simulink subsystem "TrqDemController"  (R2020b)
settings: Solver=VariableStepAuto  StartTime=0.0  StopTime=10.0  RelTol=1e-3
undefined symbols (not defined in the file): brkTrqMax, brkTrqMGU, TrqICMax, TrqMax, TrqMGUMax
libraries: eeGeneralControl x2
settings Model: Creator=francescoprignoli  LastModifiedBy=francescoprignoli

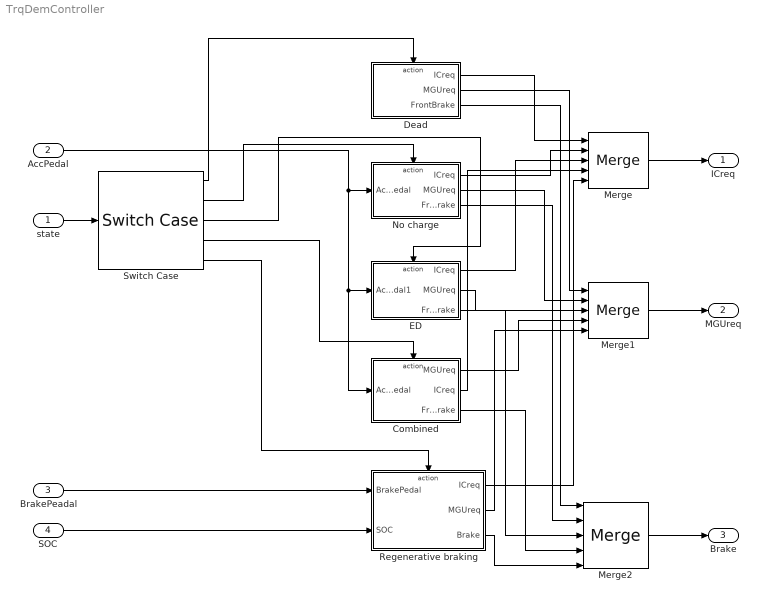
== system TrqDemController ==
  state : Inport
  AccPedal : Inport  Port=2
  BrakePeadal : Inport  Port=3
  SOC : Inport  Port=4
  Combined : Subsystem  TreatAsAtomicUnit=on
  Dead : Subsystem  TreatAsAtomicUnit=on
  ED : Subsystem  TreatAsAtomicUnit=on
  Merge : Merge  Inputs=5
  Merge1 : Merge  Inputs=5
  Merge2 : Merge  Inputs=5
  No charge : Subsystem  TreatAsAtomicUnit=on
  Regenerative braking : Subsystem  TreatAsAtomicUnit=on
  Switch Case : SwitchCase  CaseConditions={0,1,2,3,4}  ShowDefaultCase=off
  ICreq : Outport
  MGUreq : Outport  Port=2
  Brake : Outport  Port=3
  wires:
  Switch Case/1 -> Dead/Action
  ED/1(ICreq) -> Merge/3
  Merge1/1 -> MGUreq/1
  Regenerative braking/2(MGUreq) -> Merge1/5
  Dead/1(ICreq) -> Merge/1
  Regenerative braking/1(ICreq) -> Merge/5
  state/1 -> Switch Case/1
  Switch Case/5 -> Regenerative braking/Action
  AccPedal/1 -> ED/1(AccPedal1), Combined/1(AccPedal), No charge/1(AccPedal)
  Switch Case/4 -> Combined/Action
  Switch Case/3 -> ED/Action
  ED/2(MGUreq) -> Merge1/3
  SOC/1 -> Regenerative braking/2(SOC)
  Combined/1(MGUreq) -> Merge1/4
  No charge/2(MGUreq) -> Merge1/2
  Dead/2(MGUreq) -> Merge1/1
  Combined/2(ICreq) -> Merge/4
  Merge/1 -> ICreq/1
  Switch Case/2 -> No charge/Action
  No charge/1(ICreq) -> Merge/2
  BrakePeadal/1 -> Regenerative braking/1(BrakePedal)
  Dead/3(FrontBrake) -> Merge2/1
  No charge/3(FrontBrake) -> Merge2/2
  ED/3(FrontBrake) -> Merge2/3
  Combined/3(FrontBrake) -> Merge2/4
  Regenerative braking/3(Brake) -> Merge2/5
  Merge2/1 -> Brake/1

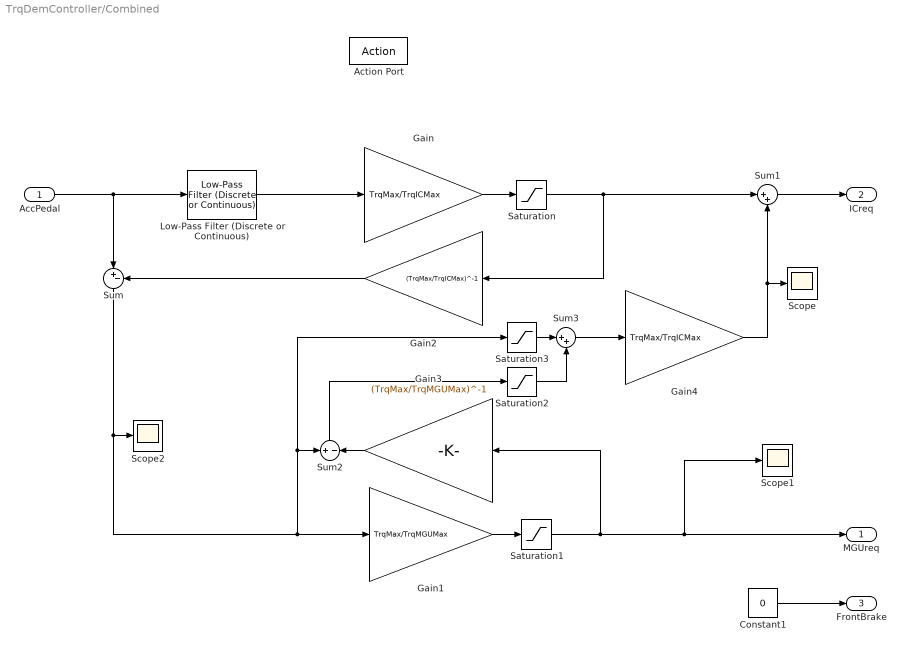
== system TrqDemController/Combined ==
  AccPedal : Inport
  Action Port : ActionPort
  Constant1 : Constant  Value=0
  Gain : Gain  Gain=TrqMax/TrqICMax
  Gain1 : Gain  Gain=TrqMax/TrqMGUMax
  Gain2 : Gain  Gain=(TrqMax/TrqICMax)^-1
  Gain3 : Gain  Gain=(TrqMax/TrqMGUMax)^-1
  Gain4 : Gain  Gain=TrqMax/TrqICMax
  Low-Pass Filter (Discrete or Continuous) : eeGeneralControl/Low-Pass Filter (Discrete or Continuous)  K=1  T=2  B=inf  A=-inf  init_option=Inherited from block input  x0=0  Ts=-1
  Saturation : Saturate  UpperLimit=1  LowerLimit=0
  Saturation1 : Saturate  UpperLimit=1  LowerLimit=0
  Saturation2 : Saturate  UpperLimit=1  LowerLimit=0
  Saturation3 : Saturate  UpperLimit=0  LowerLimit=-1
  Scope : Scope
  Scope1 : Scope
  Scope2 : Scope
  Sum : Sum  Inputs=|+-
  Sum1 : Sum  Inputs=|++
  Sum2 : Sum  Inputs=+|-
  Sum3 : Sum  Inputs=|++
  MGUreq : Outport
  ICreq : Outport  Port=2
  FrontBrake : Outport  Port=3
  wires:
  Gain4/1 -> Sum1/2, Scope/1
  Constant1/1 -> FrontBrake/1
  Saturation2/1 -> Sum3/2
  Sum3/1 -> Gain4/1
  Saturation3/1 -> Sum3/1
  Sum2/1 -> Saturation2/1
  Sum1/1 -> ICreq/1
  AccPedal/1 -> Sum/1, Low-Pass Filter (Discrete or Continuous)/1
  Sum/1 -> Sum2/1, Saturation3/1, Gain1/1, Scope2/1
  Gain/1 -> Saturation/1
  Gain1/1 -> Saturation1/1
  Saturation/1 -> Gain2/1, Sum1/1
  Saturation1/1 -> Gain3/1, MGUreq/1, Scope1/1
  Low-Pass Filter (Discrete or Continuous)/1 -> Gain/1
  Gain3/1 -> Sum2/2
  Gain2/1 -> Sum/2

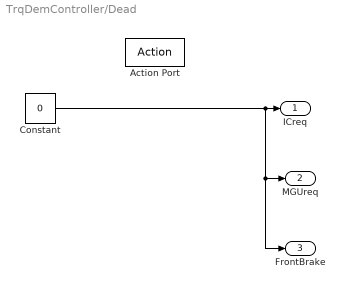
== system TrqDemController/Dead ==
  Action Port : ActionPort
  Constant : Constant  Value=0
  ICreq : Outport
  MGUreq : Outport  Port=2
  FrontBrake : Outport  Port=3
  wires:
  Constant/1 -> MGUreq/1, FrontBrake/1, ICreq/1

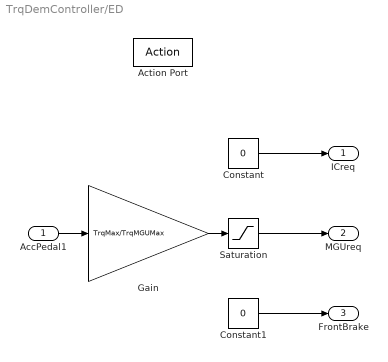
== system TrqDemController/ED ==
  AccPedal1 : Inport
  Action Port : ActionPort
  Constant : Constant  Value=0
  Constant1 : Constant  Value=0
  Gain : Gain  Gain=TrqMax/TrqMGUMax
  Saturation : Saturate  UpperLimit=1  LowerLimit=0
  ICreq : Outport
  MGUreq : Outport  Port=2
  FrontBrake : Outport  Port=3
  wires:
  Constant1/1 -> FrontBrake/1
  Constant/1 -> ICreq/1
  AccPedal1/1 -> Gain/1
  Gain/1 -> Saturation/1
  Saturation/1 -> MGUreq/1

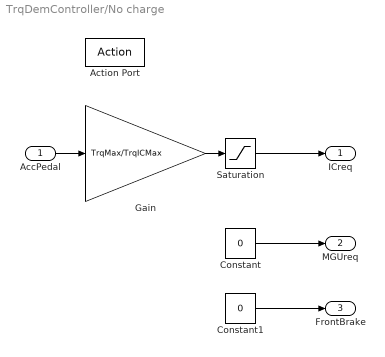
== system TrqDemController/No charge ==
  AccPedal : Inport
  Action Port : ActionPort
  Constant : Constant  Value=0
  Constant1 : Constant  Value=0
  Gain : Gain  Gain=TrqMax/TrqICMax
  Saturation : Saturate  UpperLimit=1  LowerLimit=0
  ICreq : Outport
  MGUreq : Outport  Port=2
  FrontBrake : Outport  Port=3
  wires:
  Constant1/1 -> FrontBrake/1
  Gain/1 -> Saturation/1
  AccPedal/1 -> Gain/1
  Saturation/1 -> ICreq/1
  Constant/1 -> MGUreq/1

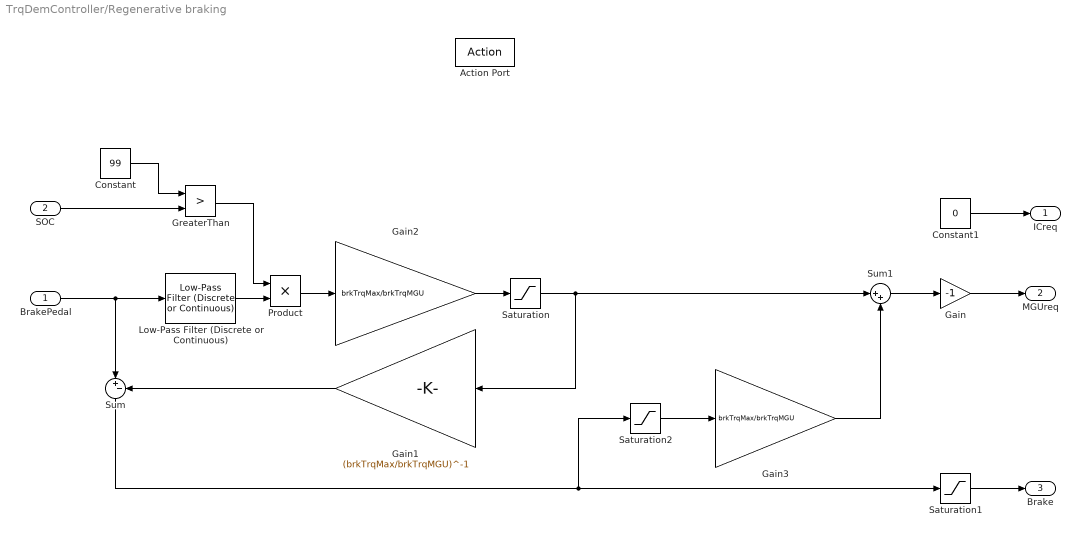
== system TrqDemController/Regenerative braking ==
  BrakePedal : Inport
  SOC : Inport  Port=2
  Action Port : ActionPort
  Constant : Constant  Value=99
  Constant1 : Constant  Value=0
  Gain : Gain  Gain=-1
  Gain1 : Gain  Gain=(brkTrqMax/brkTrqMGU)^-1
  Gain2 : Gain  Gain=brkTrqMax/brkTrqMGU
  Gain3 : Gain  Gain=brkTrqMax/brkTrqMGU
  GreaterThan : RelationalOperator  Operator=>  OutDataTypeStr=fixdt(1,16)  RndMeth=Simplest
  Low-Pass Filter (Discrete or Continuous) : eeGeneralControl/Low-Pass Filter (Discrete or Continuous)  K=1  T=1  B=inf  A=-inf  init_option=Inherited from block input  x0=0  Ts=-1
  Product : Product
  Saturation : Saturate  UpperLimit=1  LowerLimit=0
  Saturation1 : Saturate  UpperLimit=1  LowerLimit=0
  Saturation2 : Saturate  UpperLimit=0  LowerLimit=-1
  Sum : Sum  Inputs=|+-
  Sum1 : Sum  Inputs=|++
  ICreq : Outport
  MGUreq : Outport  Port=2
  Brake : Outport  Port=3
  wires:
  Sum1/1 -> Gain/1
  Gain3/1 -> Sum1/2
  Saturation2/1 -> Gain3/1
  Gain/1 -> MGUreq/1
  Constant1/1 -> ICreq/1
  Constant/1 -> GreaterThan/1
  SOC/1 -> GreaterThan/2
  Saturation1/1 -> Brake/1
  BrakePedal/1 -> Sum/1, Low-Pass Filter (Discrete or Continuous)/1
  Sum/1 -> Saturation1/1, Saturation2/1
  Gain2/1 -> Saturation/1
  Saturation/1 -> Sum1/1, Gain1/1
  Low-Pass Filter (Discrete or Continuous)/1 -> Product/2
  Product/1 -> Gain2/1
  Gain1/1 -> Sum/2
  GreaterThan/1 -> Product/1
